simulink model "IP_Arduino_implementation"  (R2023b)
settings: Solver=ode3  StartTime=0.0  StopTime=inf  RelTol=1e-3  EnableMultiTasking=on
values from neighbouring files (symbols this model uses):
  distancePerCount = 0.036    [init_param_ip.m]
  encoderCountsPerUnit = 1040    [init_param_ip.m]
libraries: arduinolib x4
settings Model: SimulationMode=external  ExtModeTrigDuration=2  Creator=mbelge  LastModifiedBy=randr
settings SolverCC: AlgebraicLoopSolver=TrustRegion
settings DataIOCC: LimitDataPoints=on  SaveFormat=Array  ReturnWorkspaceOutputs=off
settings OptimizationCC: EnhancedBackFolding=on  PassReuseOutputArgsAs=Individual arguments  ZeroExternalMemoryAtStartup=off  ZeroInternalMemoryAtStartup=off  MaxStackSize=64  OptimizeBlockOrder=speed  DifferentSizesBufferReuse=on  OptimizationCustomize=off  EfficientTunableParamExpr=on
settings DebuggingCC: UnderspecifiedInitializationDetection=Classic  MergeDetectMultiDrivingBlocksExec=none  ParameterTunabilityLossMsg=error  UnconnectedInputMsg=warning  UnconnectedOutputMsg=warning  UnconnectedLineMsg=warning  SFUnexpectedBacktrackingDiag=warning  SFNoUnconditionalDefaultTransitionDiag=warning  SFExecutionAtInitializationDiag=none  ArithmeticOperatorsInVariantConditions=warning
settings HardwareCC: ProdBitPerInt=16  ProdBitPerPointer=16  ProdBitPerSizeT=16  ProdBitPerPtrDiffT=16  ProdLargestAtomicFloat=None  ProdWordSize=8  ProdHWDeviceType=Atmel->AVR
settings ModelReferenceCC: PropagateSignalLabelsOutOfModel=off
settings SFSimCC: SimUseLocalCustomCode=off  MATLABDynamicMemAlloc=off  CustomCodeUndefinedFunction=UseInterfaceOnly
settings RTWCC: Description=Embedded Coder  SystemTargetFile=ert.tlc  HardwareBoard=Arduino Nano 3.0  TemplateMakefile=ert_default_tmf  RTWVerbose=off  RTWUseLocalCustomCode=off  Toolchain=Arduino AVR  BuildConfiguration=Faster Runs
settings CodeAppCC: ForceParamTrailComments=on  IgnoreCustomStorageClasses=off  OperatorAnnotations=on  SimulinkDataObjDesc=on  SFDataObjDesc=on  InsertBlockDesc=on
settings ERTTargetCC: SupportContinuousTime=on  SupportVariableSizeSignals=on  ExtMode=on  ExtModeTransport=3  ExtModeStaticAlloc=on  ExtModeAutomaticAllocSize=off  ExtModeStaticAllocSize=250  ExtModeMexFile=ext_xcp  ExtModeMexArgs=0 3 115200  ExtModeIntrfLevel=Level2 - Open
settings ConfigComp: CovMetricSettings=dw  CovSaveCumulativeToWorkspaceVar=on  CovSaveSingleToWorkspaceVar=on  CovExternalEMLEnable=off  CovSFcnEnable=off

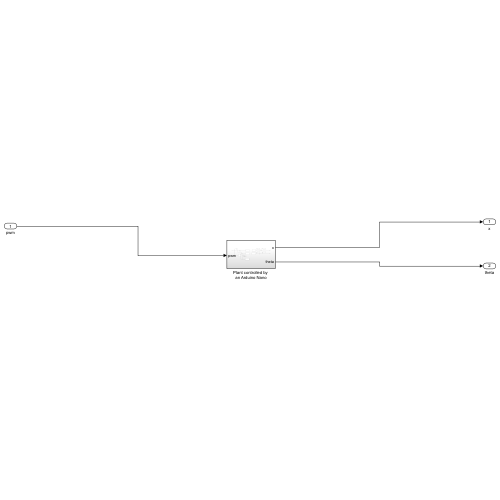
[thumbnail: Simulink's stored preview of the top-level diagram]
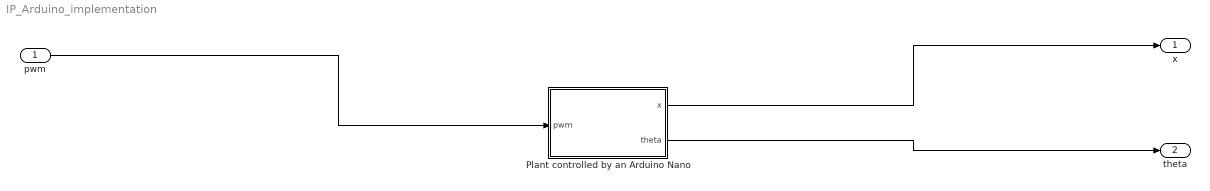
== system IP_Arduino_implementation ==
  pwm : Inport
  Plant controlled by an Arduino Nano : Subsystem
  x : Outport
  theta : Outport  Port=2
  wires:
  pwm/1 -> Plant controlled by an Arduino Nano/1(pwm)
  Plant controlled by an Arduino Nano/1(x) -> x/1
  Plant controlled by an Arduino Nano/2(theta) -> theta/1

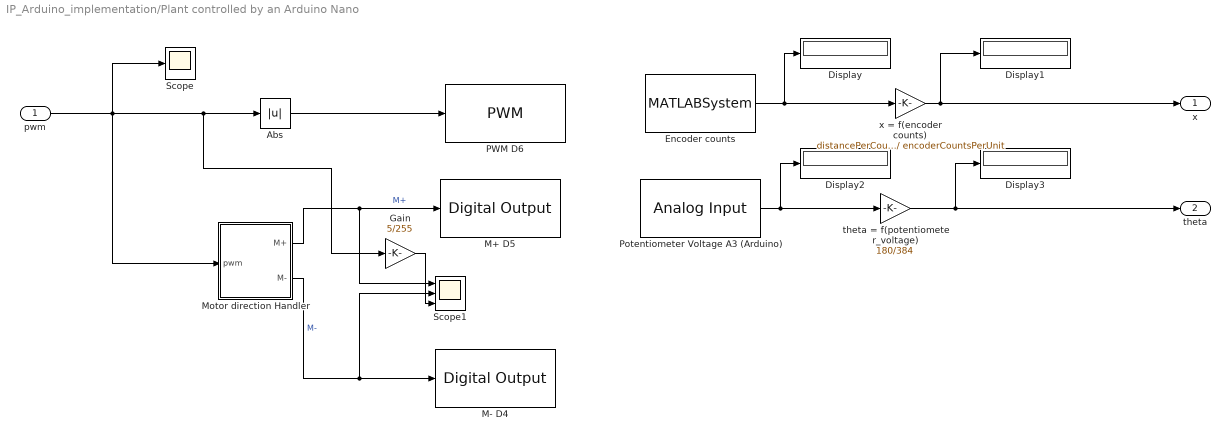
== system IP_Arduino_implementation/Plant controlled by an Arduino Nano ==
  pwm : Inport
  Abs : Abs  SaturateOnIntegerOverflow=off
  Display{,1..3} (4 alike) : Display
  Encoder counts : MATLABSystem  System=Encoder_arduino  Encoder=0  PinA=2  PinB=3  SampleTime=0.01
      mask Type: Encoder_arduino
      mask Display:
      | disp('Encoder');
      | port_label('output',1,'y');
  Gain : Gain  Gain=5/255
  M+ D5 : arduinolib/Digital Output  pinNumber=5  Direction=output  blockPlatform=arduino
  M- D4 : arduinolib/Digital Output  pinNumber=4  Direction=output  blockPlatform=arduino
  Motor direction Handler : Subsystem
  PWM D6 : arduinolib/PWM  pinNumber=6  frequencyType=Default  desiredFrequency=490.2  achievableFrequency=490.2
  Potentiometer Voltage A3 (Arduino) : arduinolib/Analog Input  pinNumber=3  ReadResultsOnly=off  ConversionTriggerSource=Software  ExternalTriggerType=uint32( 0 )  OutputDataType=uint16  EnableConversionCompleteNotify=off  EnableOuputStatus=off  SampleTime=-1  blockPlatform=arduino
  Scope : Scope
  Scope1 : Scope  NumInputPorts=3
  theta = f(potentiometer_voltage) : Gain  Gain=180/384
  x = f(encoder counts) : Gain  Gain=distancePerCount * pi * 100/ encoderCountsPerUnit
  x : Outport
  theta : Outport  Port=2
  wires:
  Motor direction Handler/2(M-) -> Scope1/2, M- D4/1  "M-"
  Encoder counts/1 -> x = f(encoder counts)/1, Display/1
  Potentiometer Voltage A3 (Arduino)/1 -> theta = f(potentiometer_voltage)/1, Display2/1
  Abs/1 -> PWM D6/1
  Motor direction Handler/1(M+) -> Scope1/1, M+ D5/1  "M+"
  pwm/1 -> Gain/1, Abs/1, Motor direction Handler/1(pwm), Scope/1
  x = f(encoder counts)/1 -> x/1, Display1/1
  theta = f(potentiometer_voltage)/1 -> theta/1, Display3/1
  Gain/1 -> Scope1/3

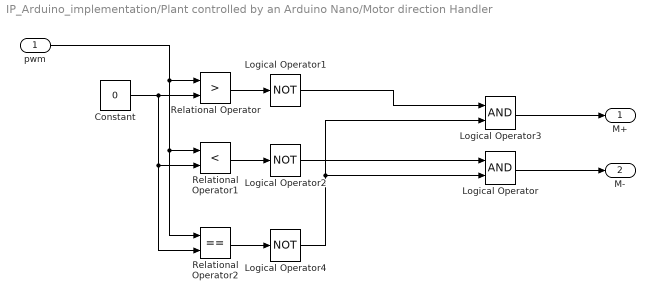
== system IP_Arduino_implementation/Plant controlled by an Arduino Nano/Motor direction Handler ==
  pwm : Inport
  Constant : Constant  Value=0
  Logical Operator : Logic  AllPortsSameDT=off  OutDataTypeStr=boolean
  Logical Operator1 : Logic  Operator=NOT  AllPortsSameDT=off  OutDataTypeStr=boolean
  Logical Operator2 : Logic  Operator=NOT  AllPortsSameDT=off  OutDataTypeStr=boolean
  Logical Operator3 : Logic  AllPortsSameDT=off  OutDataTypeStr=boolean
  Logical Operator4 : Logic  Operator=NOT  AllPortsSameDT=off  OutDataTypeStr=boolean
  Relational Operator : RelationalOperator  Operator=>  OutDataTypeStr=boolean  RndMeth=Simplest  InputSameDT=off
  Relational Operator1 : RelationalOperator  Operator=<  OutDataTypeStr=boolean  RndMeth=Simplest  InputSameDT=off
  Relational Operator2 : RelationalOperator  Operator===  OutDataTypeStr=boolean  RndMeth=Simplest  InputSameDT=off
  M+ : Outport
  M- : Outport  Port=2
  wires:
  Logical Operator4/1 -> Logical Operator3/2, Logical Operator/2
  Constant/1 -> Relational Operator2/2, Relational Operator1/2, Relational Operator/2
  Logical Operator/1 -> M-/1
  pwm/1 -> Relational Operator2/1, Relational Operator1/1, Relational Operator/1
  Logical Operator2/1 -> Logical Operator/1
  Relational Operator1/1 -> Logical Operator2/1
  Relational Operator/1 -> Logical Operator1/1
  Logical Operator1/1 -> Logical Operator3/1
  Relational Operator2/1 -> Logical Operator4/1
  Logical Operator3/1 -> M+/1
